simulink model "simulink_discrete"  (R2023b)
settings: Solver=ode45  StartTime=0.0  StopTime=0.7  RelTol=1e-3  EnableMultiTasking=on
undefined symbols (not defined in the file): Ts1, Ts2
libraries: cstblocks x2
settings Model: Creator=Koldo  LastModifiedBy=chris
settings SolverCC: AlgebraicLoopSolver=TrustRegion
settings DataIOCC: LimitDataPoints=on  SaveFormat=Array  SignalLoggingSaveFormat=ModelDataLogs  ReturnWorkspaceOutputs=off
settings OptimizationCC: ExpressionDepthLimit=2147483647  LifeSpan=inf
settings DebuggingCC: UnderspecifiedInitializationDetection=Classic  MergeDetectMultiDrivingBlocksExec=none  SolverPrmCheckMsg=warning  FcnCallInpInsideContextMsg=warning  UnconnectedInputMsg=warning  UnconnectedOutputMsg=warning  UnconnectedLineMsg=warning  StateNameClashWarn=warning  SFUnexpectedBacktrackingDiag=warning  SFNoUnconditionalDefaultTransitionDiag=warning  SFExecutionAtInitializationDiag=none  ArithmeticOperatorsInVariantConditions=warning
settings HardwareCC: ProdBitPerPointer=32  ProdBitPerSizeT=32  ProdBitPerPtrDiffT=32  ProdLargestAtomicFloat=None  ProdIntDivRoundTo=Undefined  ProdEndianess=Unspecified  ProdWordSize=32  ProdHWDeviceType=32-bit Generic
settings ModelReferenceCC: EnableRefExpFcnMdlSchedulingChecks=on  PropagateSignalLabelsOutOfModel=off
settings SFSimCC: SimUseLocalCustomCode=off  CustomCodeUndefinedFunction=UseInterfaceOnly
settings RTWCC: RTWUseLocalCustomCode=off  DLArmComputeVersion=19.05
settings CodeAppCC: StateflowObjectComments=on
settings GRTTargetCC: TargetLangStandard=C89/C90 (ANSI)  CombineOutputUpdateFcns=off  GRTInterface=on
settings ConfigComp: CovMetricSettings=dw  CovSaveCumulativeToWorkspaceVar=on  CovSaveSingleToWorkspaceVar=on  CovExternalEMLEnable=off

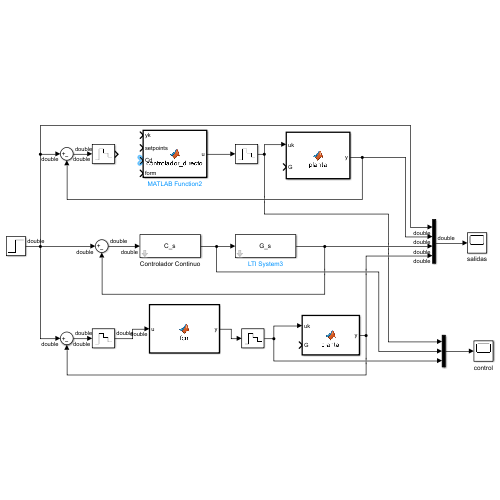
[thumbnail: Simulink's stored preview of the top-level diagram]
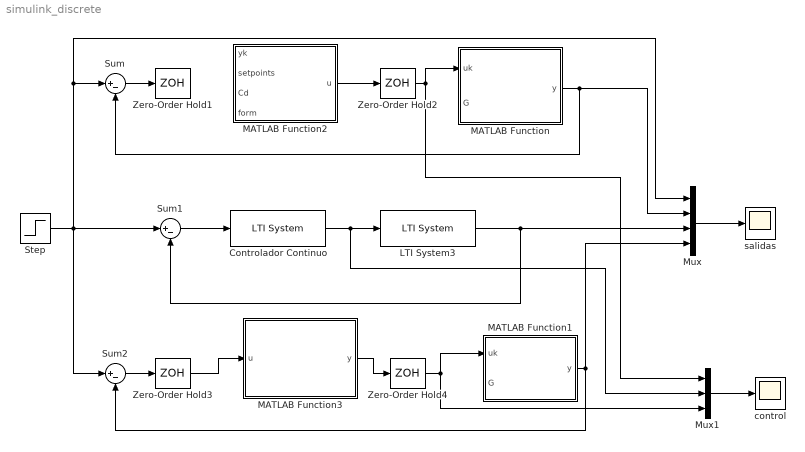
== system simulink_discrete ==
  Controlador Continuo : cstblocks/LTI System  sys=C_s  IC=[]  PadeOrder=0
  LTI System3 : cstblocks/LTI System  sys=G_s  IC=[]  PadeOrder=0
  MATLAB Function : MATLAB Function  TreatAsAtomicUnit=on
  MATLAB Function1 : MATLAB Function  TreatAsAtomicUnit=on
  MATLAB Function2 : MATLAB Function  TreatAsAtomicUnit=on
  MATLAB Function3 : MATLAB Function  TreatAsAtomicUnit=on
  Mux : Mux
  Mux1 : Mux  Inputs=3
  Step : Step  Time=0  After=pi  SampleTime=0
  Sum : Sum  Inputs=|+-
  Sum1 : Sum  Inputs=|+-
  Sum2 : Sum  Inputs=|+-
  Zero-Order Hold1 : ZeroOrderHold  SampleTime=Ts1
  Zero-Order Hold2 : ZeroOrderHold  SampleTime=-1
  Zero-Order Hold3 : ZeroOrderHold  SampleTime=Ts2
  Zero-Order Hold4 : ZeroOrderHold  SampleTime=-1
  control : Scope
  salidas : Scope
  wires:
  Sum/1 -> Zero-Order Hold1/1
  Zero-Order Hold2/1 -> Mux1/1, MATLAB Function/1(uk)
  MATLAB Function2/1(u) -> Zero-Order Hold2/1
  Step/1 -> Sum2/1, Sum1/1, Sum/1, Mux/1
  Sum1/1 -> Controlador Continuo/1
  LTI System3/1 -> Sum1/2, Mux/3
  Controlador Continuo/1 -> LTI System3/1, Mux1/2
  Mux/1 -> salidas/1
  Sum2/1 -> Zero-Order Hold3/1
  MATLAB Function1/1(y) -> Sum2/2, Mux/4
  Zero-Order Hold3/1 -> MATLAB Function3/1(u)
  MATLAB Function3/1(y) -> Zero-Order Hold4/1
  Zero-Order Hold4/1 -> MATLAB Function1/1(uk), Mux1/3
  Mux1/1 -> control/1
  MATLAB Function/1(y) -> Mux/2, Sum/2

== matlab function simulink_discrete/MATLAB Function1 ==
  data: uk input; y output; G input
function y = planta(uk, G)

%Simula el comportamiento de la planta G (LTI) en tiempo discreto

as = G.den{1,1};
bs = G.num{1,1};

%Parámetros de la planta
%a0 = as(1);
a1 = as(2);
a2 = as(3);
b0 = bs(1);
b1 = bs(2);
b2 = bs(3);

% y(k)=b0.u(k)+b1*u(k-1)+b2*u(k-2)-a1*y(k-1)-a2*y(k-2);

%Registros
persistent uk1 uk2 yk1 yk2

%Inicializamos los registros
if isempty (yk1)
    yk1=0;
end
if isempty (yk2)
    yk2=0;
end
if isempty (uk1)
    uk1=0;
end
if isempty (uk2)
    uk2=0;
end

%Cálculo de la salida de la planta
% bu0 = b0*uk;
% bu1 = b1*uk1;
% bu2 = b2*uk2;
% ay1 = a1*yk1;
% ay2 = a2*yk2;
% 
% bu01 = bu0+bu1;
% bu012 = bu01+bu2;
% ay12 = ay1+ay2;
% y = bu012 - ay12;

y=b0*uk+b1*uk1+b2*uk2-a1*yk1-a2*yk2;

%Actualizamos los registros
yk2=yk1;
yk1=y;
uk2=uk1;
uk1=uk;

function y = fcn(u)

y = u;

== matlab function simulink_discrete/MATLAB Function ==
  data: uk input; y output; G input
function y = planta(uk, G)

%Simula el comportamiento de la planta G (LTI) en tiempo discreto

as = G.den{1,1};
bs = G.num{1,1};

%Parámetros de la planta
%a0 = as(1);
a1 = as(2);
a2 = as(3);
b0 = bs(1);
b1 = bs(2);
b2 = bs(3);

% y(k)=b0.u(k)+b1*u(k-1)+b2*u(k-2)-a1*y(k-1)-a2*y(k-2);

%Registros
persistent uk1 uk2 yk1 yk2

%Inicializamos los registros
if isempty (yk1)
    yk1=0;
end
if isempty (yk2)
    yk2=0;
end
if isempty (uk1)
    uk1=0;
end
if isempty (uk2)
    uk2=0;
end

%Cálculo de la salida de la planta
% bu0 = b0*uk;
% bu1 = b1*uk1;
% bu2 = b2*uk2;
% ay1 = a1*yk1;
% ay2 = a2*yk2;
% 
% bu01 = bu0+bu1;
% bu012 = bu01+bu2;
% ay12 = ay1+ay2;
% y = bu012 - ay12;

y=b0*uk+b1*uk1+b2*uk2-a1*yk1-a2*yk2;

%Actualizamos los registros
yk2=yk1;
yk1=y;
uk2=uk1;
uk1=uk;

== matlab function simulink_discrete/MATLAB Function2 ==
  data: yk input; u output; setpoints input; Cd input; form input

function u = controlador_directo(yk, setpoints, Cd,form)
%C_s= tf([0.0050,1,0],[0.5250,5.0220,4.4000])

global ek;
% Simula el cálculo de la señal de control del controlador C en tiempo
% discreto. Implementación directa 1D.
% Entradas:
% yk: estado de la planta (posición)
% setpoints: Valor del setpoint (referencia)
% Cd: FT del controlador discretizado
% form: forma directa (1D, 2D, 3D, 4D)

% Extraemos los valores de los parámetros del controlador
as = C_s.den{1,1};
bs = C_s.num{1,1};

%Parámetros del controlador
%a0 = as(1);
a1 = as(2);
a2 = as(3);
b0 = bs(1);
b1 = bs(2);
b2 = bs(3);

% Registros 1D
persistent pk1 pk2
% Registros 2D
persistent q1k1 q2k1
% Registros 3D
persistent ek1 ek2 uk1 uk2
% Registros 4D
persistent  p0k1 p1k1 p2k1

% Selección de la realización (estructura)
if strcmp(form,'1D')
    % Forma canónica (2 registros). Sensible a la cuantificación numérica.
    % uk = b0(ek-a1*pk1-a2*pk2) + b1*pk1 + b2*pk2;
    % Inicializamos los registros (reset)
    if isempty (pk1)
        pk1=0;
    end
    if isempty (pk2)
        pk2=0;
    end
    
    %Realimentación
    ek = setpoints - yk;
    
    %Cálculo de la señal de control
    apk1 = a1*pk1;
    apk2 = a2*pk2;
    pk = ek - apk1 - apk2;
    
    bpk = b0*pk;
    bpk1 = b1*pk1;
    bpk2 = b2*pk2;
    uk = bpk + bpk1 + bpk2;
    
    %Actualizamos los registros
    pk2=pk1;
    pk1=pk;
    u=uk;
    
elseif strcmp(form,'2D')
    % Canónica. Dos registros.
    % u(k)  = b0*e(k) + q1(k-1)
    % q1(k) = q2(k-1) + b1*e(k) - a1*u(k)
    % q2(k) = b2*e(k) - a2*u(k)

    if isempty (q1k)
        q1k=0;
    end
    if isempty (q2k)
        q2k=0;
    end

     if isempty (q1k1)
        q1k1=0;
     end
       if isempty (q2k1)
        q2k1=0;
     end
    ek = setpoints -yk;
    
    u = b0*ek + q1k1;

    q2k = b2*ek-a2*u;

    q1k = q2k1 + b1*ek - a1*u;
    
    q1k1=q1k;

    q2k1=q2k;
    

elseif strcmp(form,'3D')
    % No canónica: cuatro registros
    % u(k) = b0*e(k)+b1*e(k-1)+b2*e(k-2)-a1*u(k-1)-a2*u(k-2)
    
     if isempty (u)
        u=0;
     end 
    if isempty (uk1)
        uk1=0;
     end
     if isempty (uk2)
        uk2=0;
    end
    if isempty (ek1)
        ek1=0;
    end
    if isempty (ek2)
        ek2=0;
    end

    ek= setpoints-u;
    u = b0*ek+b1*ek1+b2*ek2-a1*uk1-a2*uk2;
    uk2=uk1;
    uk1=u;
    ek2=ek1;
    ek1=ek;

elseif strcmp(form,'4D')
 
    if isempty (p1k1)
        p1k1=0;
    end
    if isempty (p2k1)
        p2k1=0;
    end
    if isempty (q1k1)
        q1k1=0;
    end
    if isempty (q2k1)
        q2k1=0;
    end
    if isempty (u)
        u=0;
    end
    
    ek= setpoints-u;
    p0k= ek +p1k1;
    u= p0k*bo+q1k1;
    q1k=q2k1+b1*p0k;
    q2k=p0k*b2;
    p2k=-a2*p0k;
    p1k=-a1*p0k+p2k1;
    p2k1=p2k;
    p1k1=p1k;
    q1k1=q1k;
    q2k1=q2k;   
end

== matlab function simulink_discrete/MATLAB Function3 ==
  data: u input; y output
function y = fcn(u)

y = u;

function u = controlador_directo(yk, setpoints, Cd, form)
C_s= tf([0.0050,1,0],[0.5250,5.0220,4.4000])

global ek;
% Simula el cálculo de la señal de control del controlador C en tiempo
% discreto. Implementación directa 1D.
% Entradas:
% yk: estado de la planta (posición)
% setpoints: Valor del setpoint (referencia)
% Cd: FT del controlador discretizado
% form: forma directa (1D, 2D, 3D, 4D)

% Extraemos los valores de los parámetros del controlador
as = C_s.den{1,1};
bs = C_s.num{1,1};

%Parámetros del controlador
%a0 = as(1);
a1 = as(2);
a2 = as(3);
b0 = bs(1);
b1 = bs(2);
b2 = bs(3);

% Registros 1D
persistent pk1 pk2
% Registros 2D
persistent q1k1 q2k1
% Registros 3D
persistent ek1 ek2 uk1 uk2
% Registros 4D
persistent  p0k1 p1k1 p2k1

% Selección de la realización (estructura)
if strcmp(form,'1D')
    % Forma canónica (2 registros). Sensible a la cuantificación numérica.
    % uk = b0(ek-a1*pk1-a2*pk2) + b1*pk1 + b2*pk2;
    % Inicializamos los registros (reset)
    if isempty (pk1)
        pk1=0;
    end
    if isempty (pk2)
        pk2=0;
    end
    
    %Realimentación
    ek = setpoints - yk;
    
    %Cálculo de la señal de control
    apk1 = a1*pk1;
    apk2 = a2*pk2;
    pk = ek - apk1 - apk2;
    
    bpk = b0*pk;
    bpk1 = b1*pk1;
    bpk2 = b2*pk2;
    uk = bpk + bpk1 + bpk2;
    
    %Actualizamos los registros
    pk2=pk1;
    pk1=pk;
    u=uk;
    
elseif strcmp(form,'2D')
    % Canónica. Dos registros.
    % u(k)  = b0*e(k) + q1(k-1)
    % q1(k) = q2(k-1) + b1*e(k) - a1*u(k)
    % q2(k) = b2*e(k) - a2*u(k)

    if isempty (q1k)
        q1k=0;
    end
    if isempty (q2k)
        q2k=0;
    end

     if isempty (q1k1)
        q1k1=0;
     end
       if isempty (q2k1)
        q2k1=0;
     end
    ek = setpoints -yk;
    
    u = b0*ek + q1k1;

    q2k = b2*ek-a2*u;

    q1k = q2k1 + b1*ek - a1*u;
    
    q1k1=q1k;

    q2k1=q2k;
    

elseif strcmp(form,'3D')
    % No canónica: cuatro registros
    % u(k) = b0*e(k)+b1*e(k-1)+b2*e(k-2)-a1*u(k-1)-a2*u(k-2)
    
     if isempty (u)
        u=0;
     end 
    if isempty (uk1)
        uk1=0;
     end
     if isempty (uk2)
        uk2=0;
    end
    if isempty (ek1)
        ek1=0;
    end
    if isempty (ek2)
        ek2=0;
    end

    ek= setpoints-u;
    u = b0*ek+b1*ek1+b2*ek2-a1*uk1-a2*uk2;
    uk2=uk1;
    uk1=u;
    ek2=ek1;
    ek1=ek;

elseif strcmp(form,'4D')
 
    if isempty (p1k1)
        p1k1=0;
    end
    if isempty (p2k1)
        p2k1=0;
    end
    if isempty (q1k1)
        q1k1=0;
    end
    if isempty (q2k1)
        q2k1=0;
    end
    if isempty (u)
        u=0;
    end
    
    ek= setpoints-u;
    p0k= ek +p1k1;
    u= p0k*bo+q1k1;
    q1k=q2k1+b1*p0k;
    q2k=p0k*b2;
    p2k=-a2*p0k;
    p1k=-a1*p0k+p2k1;
    p2k1=p2k;
    p1k1=p1k;
    q1k1=q1k;
    q2k1=q2k;   
end
